simulink model "RoboBoatVU_2014_Bacchus"  (R2014a)
settings: Solver=FixedStepDiscrete  StartTime=0.0  StopTime=inf  FixedStep=.1  RelTol=1e-3
undefined symbols (not defined in the file): Com1, Com2, Com3, Com4, DiscIntNeverNeededParam, RGB24, standard
libraries: visiontextngfix x51, simulink x44, xpcseriallib x15, dspmtrx3 x14, speedgoatlib_IO102 x3, slrtlib x2, visionstatistics x2, dspstat3 x2, dspindex x2, xpcvideousblib x2, xpcvideoutillib x2, speedgoatlib x1
(part 2 of 5)

== matlab function RoboBoatVU_2014_Bacchus/Main FSM/Obstacle Navigation1/Enter Gate/Gate 1 (Red & White)/Distance ==
  data: Distance output; DesiredGPS input; GPSLat input; GPSLong input
function Distance  = DistCalc(DesiredGPS, GPSLat, GPSLong)

%Written by Anderson Lebbad on July 22, 2013
%Last Edited:

%Orients the boat towards a target GPS point before approaching it.
%This is done to keep the approach angle minimal, so the approach
%algorithm does not circle the target and never reach it.

%Parse input GPS and convert angles to radians
CurLat = (floor(GPSLat/100)+mod(GPSLat,100)/60)*pi/180;
CurLong = (floor(GPSLong/100)+mod(GPSLong,100)/60)*pi/180;
DesLat = (floor(DesiredGPS(1)/100)+mod(DesiredGPS(1),100)/60)*pi/180;
DesLong = (floor(DesiredGPS(2)/100)+mod(DesiredGPS(2),100)/60)*pi/180;
%Difference between lats and longs
DiffLat = DesLat - CurLat;
MidLat = cos((CurLat + DesLat)/2);
DiffLong = DesLong - CurLong;
%Radius of the earth in meters
R = 6378137;

%Calculate distance using the great-circle distance formula
%Formula documented here:
%   http://www.movable-type.co.uk/scripts/latlong.html
% a = sin(DiffLat/2)^2+sin(DiffLong/2)^2*cos(CurLat)*cos(DesLat);
% c = 2*atan2(sqrt(a), sqrt(1-a));
% Distance = R*c;

%Calculating distance using Pythagora's
a = DiffLong*MidLat;
b = DiffLat;
Distance = R*sqrt(a^2+b^2);

== matlab function RoboBoatVU_2014_Bacchus/Main FSM/Obstacle Navigation1/Enter Gate/Gate 2 (White & White)/MATLAB Function ==
  data: Prob input; RPM output; ColorID input; Dist input; Ang input; CurrentHeading input; GPSLat input; GPSLong input; Timer input; DesiredHeading output; gateGPS output
function [RPM,DesiredHeading,gateGPS] = navigation(Prob,ColorID,Dist,Ang,CurrentHeading,GPSLat,GPSLong,Timer)

% Function performs one buoy navigation through the start speed gates. If
% no buoys are found by the LIDAR/Vision assembly then an incremented
% turning algorithm is executed to turn by 10 degrees per increment up to 
% 90 degrees either way of the inital heading

% Written by Edward Zhu


persistent LockHeading TimeLastFound Counter Turn TurnInc gateLat gateLong

if isempty(LockHeading) && isempty(TimeLastFound) && isempty(Counter) && isempty(Turn) && isempty(TurnInc)
    LockHeading = CurrentHeading;
    TimeLastFound = 0;
    Counter = 0;
    TurnInc = 30;
    Turn = TurnInc;
    gateLat = 0;
    gateLong = 0;
end
Distance = Dist/100;
BoatWidth = 0.75;
Buffer = atan(2*BoatWidth/Distance);

RedOffset = Ang + Buffer;
WhiteOffset = Ang - Buffer;

R = 6378137;

CurLat = (floor(GPSLat/100)+mod(GPSLat,100)/60)*pi/180;
CurLong = (ceil(GPSLong/100)-mod(-GPSLong,100)/60)*pi/180;

gateHeading = (mod(CurrentHeading - Ang, 360))*pi/180;

if ColorID == 1 && Prob > 0.9
    DesiredHeading = mod(CurrentHeading - RedOffset, 360);
    RPM = 2000;
    GateFound = 1;
    TimeLastFound = Timer;
    gateLat =  asin(sin(CurLat)*cos(Distance/R) + cos(CurLat)*sin(Distance/R)*cos(gateHeading))*180/pi;
    gateLong = (CurLong + atan2(sin(gateHeading)*sin(Distance/R)*cos(CurLat),cos(Distance/R)-sin(CurLat)*sin(gateLat)))*180/pi;
elseif ColorID == 2 && Prob > 0.9
    DesiredHeading = mod(CurrentHeading - WhiteOffset, 360);
    RPM = 2000;
    GateFound = 1;
    TimeLastFound = Timer;
    gateLat =  asin(sin(CurLat)*cos(Distance/R) + cos(CurLat)*sin(Distance/R)*cos(gateHeading))*180/pi;
    gateLong = (CurLong + atan2(sin(gateHeading)*sin(Distance/R)*cos(CurLat),cos(Distance/R)-sin(CurLat)*sin(gateLat)))*180/pi;
else
    DesiredHeading = CurrentHeading;
    RPM = 0;
    GateFound = 0;
end

gateGPS = [gateLat gateLong];
TimeNoBuoys = Timer - TimeLastFound;

if GateFound == 0 && TimeNoBuoys > 15
    RPM = 0;
    DesiredHeading = mod(LockHeading - Turn, 360);
    HeadingDiff = DesiredHeading - CurrentHeading;
    gateGPS = [gateLat gateLong];
    
    if HeadingDiff > 180
        HeadingDiff = HeadingDiff - 360;
    elseif HeadingDiff < -180
        HeadingDiff = HeadingDiff + 360;
    end
    
    if HeadingDiff < 3
        Counter = Counter + 1;
    else
        Counter = 0;
    end
    
    if Counter >= 15
        Turn = Turn + TurnInc;
        Counter = 0;
        if abs(Turn) > 90
            TurnInc = -TurnInc;
        end
    end
end

== matlab function RoboBoatVU_2014_Bacchus/Main FSM/Communication/Docking Bay Comm/MATLAB Function ==
  data: requestNumOut output; CP input; requestNumIn input; Finished output
function [requestNumOut, Finished] = requestSender(CP, requestNumIn)

if CP < 1
    requestNumOut = requestNumIn;
    Finished = 0;
else
    requestNumOut = 0;
    Finished = 1;
end
end

== matlab function RoboBoatVU_2014_Bacchus/Main FSM/Color Sequence Detection/Report/MATLAB Function ==
  data: requestNumOut output; CP input; requestNumIn input; Finished output
function [requestNumOut, Finished] = requestSender(CP, requestNumIn)

if CP < 1
    requestNumOut = requestNumIn;
    Finished = 0;
else
    requestNumOut = 0;
    Finished = 1;
end

== matlab function RoboBoatVU_2014_Bacchus/Main FSM/Obstacle Navigation1/GPS: Center/Approach/Desired Heading and Distance ==
  data: Distance output; DesiredGPS input; DesiredHeading output; GPSLat input; GPSLong input
function [Distance, DesiredHeading] = Approach(DesiredGPS, GPSLat, GPSLong)

%Written by Anderson Lebbad on July 22, 2013
%Last Edited: Edward Zhu July 5, 2014

%Edit:
% Switched from great-circle distance formula to equirectangular approx and
%used mod for desired heading
% Changed calculation to use positve lat and negative long

%Orients the boat towards a target GPS point before approaching it.
%This is done to keep the approach angle minimal, so the approach
%algorithm does not circle the target and never reach it.

%Parse input GPS and convert angles to radians
CurLat = (floor(GPSLat/100)+mod(GPSLat,100)/60)*pi/180;
CurLong = (ceil(GPSLong/100)-mod(-GPSLong,100)/60)*pi/180;
DesLat = (floor(DesiredGPS(1)/100)+mod(DesiredGPS(1),100)/60)*pi/180;
DesLong = (ceil(DesiredGPS(2)/100)-mod(-DesiredGPS(2),100)/60)*pi/180;

%Difference between lats and longs
DiffLat = DesLat - CurLat;
MidLat = cos((CurLat + DesLat)/2);
DiffLong = DesLong - CurLong;

%Radius of the earth in meters
R = 6378137;

%Calculate distance using the great-circle distance formula
%Formula documented here:
%   http://www.movable-type.co.uk/scripts/latlong.html
% a = sin(DiffLat/2)^2+sin(DiffLong/2)^2*cos(CurLat)*cos(DesLat);
% c = 2*atan2(sqrt(a), sqrt(1-a));
% Distance = R*c;

%Calculating distance using equirectangular approximation since distances
%concerned are very small
a = DiffLong*MidLat;
b = DiffLat;
Distance = R*sqrt(a^2+b^2);

%Calculate initial bearing - formula documented here: 
%   http://www.movable-type.co.uk/scripts/latlong.html
y = sin(DiffLong)*cos(DesLat);
x = cos(CurLat)*sin(DesLat)-sin(CurLat)*cos(DesLat)*cos(DiffLong);
DesiredHeading = mod(atan2(y, x)*180/pi + 360, 360);

== matlab function RoboBoatVU_2014_Bacchus/Main FSM/Obstacle Navigation1/Obstacle Navigation/GPS: Bee Line/Approach/Obstacle Distance ==
  data: ColorID input; ObstDist output; DodgeStart output; Dist input
function [ObstDist, DodgeStart] = obstDist(ColorID,Dist)

%Written by Edward Zhu
%Last Edited by:

ObstDist = Dist / 100;

% if ColorID == 5 || ColorID == 6
    if ObstDist <= 3
        DodgeStart = 1;
    else
        DodgeStart = 0;
    end
% else
%     DodgeStart = 0;
% end

== matlab function RoboBoatVU_2014_Bacchus/Sensors/Serial In/Decode Compass/Correct Heading Angle Magnetic to True North/Magnetic to True North Conversion ==
  data: HeadingM input; HeadingT output; MagDec input
function HeadingT = fcn(HeadingM,MagDec)
% This function corrects the compass heading reading from magnetic north to
% true north

% Magnetic declination at Villanova is -12.116 degrees (West)
% Magnetic declination at competition site is -10.877 degrees (West)

% Current physical orientation of the compass is 0 degrees north measuring
% heading CCW, the standard for measuring heading is 0 degrees north 
% measuring CW. Therefore, first the heading is corrected to true heading
% by adding the declination. Then the heading is negated and added to 360
% in order to match with the standard measurment.

HeadingT = mod((HeadingM - MagDec) + 360, 360);

== matlab function RoboBoatVU_2014_Bacchus/Main FSM/Obstacle Navigation1/Obstacle Navigation/MATLAB Function ==
  data: dodgeIncomplete input; dodgeStart input; taskSelector output; dodgeEn output; GPSEn output
function [taskSelector, dodgeEn, GPSEn]  = obstNavEnabler(dodgeIncomplete, dodgeStart)

GPSEn = 0;
dodgeEn = 0;

if  dodgeStart == 1 || dodgeIncomplete == 1
    dodgeEn = 1;
    taskSelector = 1;
else
    GPSEn = 1;
    taskSelector = 2;
end

== matlab function RoboBoatVU_2014_Bacchus/Main FSM/Main Task Option/Message Composer ==
  data: taskStrInit input; taskStrAdj output
function taskStrAdj = composeMessage(taskStrInit)
%Written by Anderson Lebbad on August 9, 2013
%Last Edited: Edward Zhu on June 2, 2014

%This function adjusts the length of a vector to a set value by filling
%the remaining space with 0's. This is necessary for data store objects
%that have a fixed size for the memory allocation, but a variable length
%input.

%Length of message packet
strLength = 8;

%Size of text in message
taskStrLength = size(taskStrInit,1);

%Pad end of text with zeros
taskStrAdj = [taskStrInit' zeros(1,strLength-taskStrLength)];

== system RoboBoatVU_2014_Bacchus/Main FSM/Communication/Docking Bay Comm ==
  Sensors : Inport
  RGB image : Inport  Port=2
  Enable : EnablePort  ShowOutputPort=on
  Annotate Task : visiontextngfix/Insert Text  inputType=Obsolete  theText='Docking Bay Request...'  getTextLocFrom=Specify via dialog  textLoc=[10 10]  getTextColorFrom=Specify via dialog  textColor=[0 0 255]  getTextIntensityFrom=Specify via dialog  textIntensity=0  getTextOpacityFrom=Specify via dialog  textOpacity=1.0  dummyVar2=0  dummyVar3=0  dummyVar4=0  imagePorts=One multidimensional signal  isInputTransposed=off  fontFace=LucidaSansRegular  dummyVar1=0  blockFontSize=12  antiAliased=on
  Annotate Task1 : visiontextngfix/Insert Text  inputType=Obsolete  theText='CP: %f'  getTextLocFrom=Specify via dialog  textLoc=[10 20]  getTextColorFrom=Specify via dialog  textColor=[0 0 255]  getTextIntensityFrom=Specify via dialog  textIntensity=0  getTextOpacityFrom=Specify via dialog  textOpacity=1.0  dummyVar2=0  dummyVar3=0  dummyVar4=0  imagePorts=One multidimensional signal  isInputTransposed=off  fontFace=LucidaSansRegular  dummyVar1=0  blockFontSize=12  antiAliased=on
  Bus Selector : BusSelector  OutputSignals=Serial In.Compass.Heading,Serial In.Comms.CP,Serial In.Comms.Dat1
  Compare To Constant : simulink/Logic and Bit Operations/Compare To Constant  relop=>=  const=15  OutDataTypeStr=boolean
  Constant : Constant  Value=2
  Data Store Write : DataStoreWrite  DataStoreName=dockBay
  Data Type Conversion : DataTypeConversion  OutDataTypeStr=double
  Discrete-Time Integrator : DiscreteIntegrator  SampleTime=0.1  ICPrevOutput=DiscIntNeverNeededParam  ICPrevScaledInput=DiscIntNeverNeededParam
  Logical Operator : Logic  Operator=OR  AllPortsSameDT=off  OutDataTypeStr=boolean
  MATLAB Function : MATLAB Function  TreatAsAtomicUnit=on
  Output Heirarchy : Subsystem
  Outputs : Outport
  wires:
  Sensors/1 -> Bus Selector/1, Output Heirarchy/3(Sensors)  "Sensors"
  Bus Selector/1 -> Output Heirarchy/2(Desired Heading)  "<Heading>"
  RGB image/1 -> Annotate Task/1
  Annotate Task/1 -> Annotate Task1/1
  Output Heirarchy/1(Outputs) -> Outputs/1
  Enable/1 -> Discrete-Time Integrator/1
  Discrete-Time Integrator/1 -> Compare To Constant/1
  Data Type Conversion/1 -> Output Heirarchy/5(Task Finished)
  Bus Selector/2 -> Annotate Task1/2, MATLAB Function/1(CP)  "<CP>"
  Constant/1 -> MATLAB Function/2(requestNumIn)
  MATLAB Function/1(requestNumOut) -> Output Heirarchy/4(Request Number)
  Logical Operator/1 -> Data Type Conversion/1
  MATLAB Function/2(Finished) -> Logical Operator/1
  Compare To Constant/1 -> Logical Operator/2
  Annotate Task1/1 -> Output Heirarchy/1(Annotated Image)
  Bus Selector/3 -> Data Store Write/1  "<Dat1>"

== system RoboBoatVU_2014_Bacchus/Main FSM/Communication/Obst Gate Comm ==
  Sensors : Inport
  RGB image : Inport  Port=2
  Enable : EnablePort  ShowOutputPort=on
  Annotate Task : visiontextngfix/Insert Text  inputType=Obsolete  theText='Obstacle Navigation Request...'  getTextLocFrom=Specify via dialog  textLoc=[10 10]  getTextColorFrom=Specify via dialog  textColor=[0 0 255]  getTextIntensityFrom=Specify via dialog  textIntensity=0  getTextOpacityFrom=Specify via dialog  textOpacity=1.0  dummyVar2=0  dummyVar3=0  dummyVar4=0  imagePorts=One multidimensional signal  isInputTransposed=off  fontFace=LucidaSansRegular  dummyVar1=0  blockFontSize=12  antiAliased=on
  Annotate Task1 : visiontextngfix/Insert Text  inputType=Obsolete  theText='CP: %f'  getTextLocFrom=Specify via dialog  textLoc=[10 20]  getTextColorFrom=Specify via dialog  textColor=[0 0 255]  getTextIntensityFrom=Specify via dialog  textIntensity=0  getTextOpacityFrom=Specify via dialog  textOpacity=1.0  dummyVar2=0  dummyVar3=0  dummyVar4=0  imagePorts=One multidimensional signal  isInputTransposed=off  fontFace=LucidaSansRegular  dummyVar1=0  blockFontSize=12  antiAliased=on
  Bus Selector : BusSelector  OutputSignals=Serial In.Comms.CP,Serial In.Comms.Dat1,Serial In.Comms.Dat2,Serial In.Compass.Heading
  Compare To Constant : simulink/Logic and Bit Operations/Compare To Constant  relop=>=  const=15  OutDataTypeStr=boolean
  Constant : Constant
  Data Store Write : DataStoreWrite  DataStoreName=enterGate
  Data Store Write1 : DataStoreWrite  DataStoreName=exitGate
  Data Type Conversion : DataTypeConversion  OutDataTypeStr=double
  Discrete-Time Integrator : DiscreteIntegrator  SampleTime=0.1  ICPrevOutput=DiscIntNeverNeededParam  ICPrevScaledInput=DiscIntNeverNeededParam
  Logical Operator : Logic  Operator=OR  AllPortsSameDT=off  OutDataTypeStr=boolean
  MATLAB Function : MATLAB Function  TreatAsAtomicUnit=on
  Output Heirarchy : Subsystem
  Outputs : Outport
  Finished : Outport  Port=2
  wires:
  Sensors/1 -> Bus Selector/1, Output Heirarchy/3(Sensors)  "Sensors"
  Bus Selector/4 -> Output Heirarchy/2(Desired Heading)  "<Heading>"
  RGB image/1 -> Annotate Task/1
  Output Heirarchy/1(Outputs) -> Outputs/1
  Enable/1 -> Discrete-Time Integrator/1
  Discrete-Time Integrator/1 -> Compare To Constant/1
  Annotate Task/1 -> Annotate Task1/1
  Bus Selector/1 -> MATLAB Function/1(CP), Annotate Task1/2  "<CP>"
  Annotate Task1/1 -> Output Heirarchy/1(Annotated Image)
  Data Type Conversion/1 -> Finished/1
  MATLAB Function/1(requestNumOut) -> Output Heirarchy/4(Request Number)
  Constant/1 -> MATLAB Function/2(requestNumIn)
  Logical Operator/1 -> Data Type Conversion/1
  MATLAB Function/2(Finished) -> Logical Operator/1
  Compare To Constant/1 -> Logical Operator/2
  Bus Selector/2 -> Data Store Write/1  "<Dat1>"
  Bus Selector/3 -> Data Store Write1/1  "<Dat2>"

== system RoboBoatVU_2014_Bacchus/Main FSM/Communication/Output Reassign ==
  Outputs in : Inport
  Bus Selector : BusSelector  OutputSignals=Task Finished,Output Signals
  Outputs : Outport
  Finished : Outport  Port=2
  wires:
  Outputs in/1 -> Bus Selector/1
  Bus Selector/1 -> Finished/1  "<Task Finished>"
  Bus Selector/2 -> Outputs/1  "<Output Signals>"

== system RoboBoatVU_2014_Bacchus/Main FSM/Docking/Output Heirarchy ==
  Annotated Image : Inport
  Desired Heading : Inport  Port=2
  Sensors : Inport  Port=3
  Request Number : Inport  Port=4
  Bus Creator : BusCreator  Inputs=2
  Bus Creator1 : BusCreator  Inputs=3
  Bus Creator2 : BusCreator  Inputs=2
  Bus Creator3 : BusCreator  Inputs=6
  Bus Creator4 : BusCreator  Inputs=2
  C1 : Constant  Value=0
  C2 : Constant  Value=0
  C3 : Constant  Value=0
  LPTask : Constant  Value=0
  Latitude : Constant  Value=0
  Longitude : Constant  Value=0
  RPM Desired : Constant  Value=0
  Outputs : Outport
  wires:
  RPM Desired/1 -> Bus Creator/1  "RPM"
  Bus Creator/1 -> Bus Creator1/1  "Control Signals"
  Bus Creator3/1 -> Bus Creator2/1  "Comms Panda"
  Request Number/1 -> Bus Creator3/1  "Request Number"
  Latitude/1 -> Bus Creator3/2  "Latitude"
  Longitude/1 -> Bus Creator3/3  "Longitude"
  C1/1 -> Bus Creator3/4  "C1"
  LPTask/1 -> Bus Creator2/2  "LIDAR Panda"
  Desired Heading/1 -> Bus Creator/2  "Desired Heading"
  Bus Creator1/1 -> Bus Creator4/1  "Outputs"
  Annotated Image/1 -> Bus Creator1/3  "Annotated Image"
  Sensors/1 -> Bus Creator4/2  "Sensors"
  Bus Creator4/1 -> Outputs/1  "Output Signals"
  Bus Creator2/1 -> Bus Creator1/2  "Serial Outputs"
  C2/1 -> Bus Creator3/5  "C2"
  C3/1 -> Bus Creator3/6  "C3"

== system RoboBoatVU_2014_Bacchus/Main FSM/Initialization1/Output Heirarchy ==
  Annotated Image : Inport
  Desired Heading : Inport  Port=2
  Sensors : Inport  Port=3
  Request Number : Inport  Port=4
  Bus Creator : BusCreator  Inputs=2
  Bus Creator1 : BusCreator  Inputs=3
  Bus Creator2 : BusCreator  Inputs=2
  Bus Creator3 : BusCreator  Inputs=6
  Bus Creator4 : BusCreator  Inputs=2
  C1 : Constant  Value=0
  C2 : Constant  Value=0
  C3 : Constant  Value=0
  LPTask : Constant  Value=0
  Latitude : Constant  Value=0
  Longitude : Constant  Value=0
  RPM Desired : Constant  Value=0
  Outputs : Outport
  wires:
  RPM Desired/1 -> Bus Creator/1  "RPM"
  Bus Creator/1 -> Bus Creator1/1  "Control Signals"
  Bus Creator3/1 -> Bus Creator2/1  "Comms Panda"
  Request Number/1 -> Bus Creator3/1  "Request Number"
  Latitude/1 -> Bus Creator3/2  "Latitude"
  Longitude/1 -> Bus Creator3/3  "Longitude"
  C1/1 -> Bus Creator3/4  "C1"
  LPTask/1 -> Bus Creator2/2  "LIDAR Panda"
  Desired Heading/1 -> Bus Creator/2  "Desired Heading"
  Bus Creator1/1 -> Bus Creator4/1  "Outputs"
  Annotated Image/1 -> Bus Creator1/3  "Annotated Image"
  Sensors/1 -> Bus Creator4/2  "Sensors"
  Bus Creator4/1 -> Outputs/1  "Output Signals"
  Bus Creator2/1 -> Bus Creator1/2  "Serial Outputs"
  C2/1 -> Bus Creator3/5  "C2"
  C3/1 -> Bus Creator3/6  "C3"

== system RoboBoatVU_2014_Bacchus/Main FSM/Obstacle Navigation/Dodge ==
  Sensors : Inport
  RGB image : Inport  Port=2
  Enable : EnablePort  ShowOutputPort=on
  Bus Selector1 : BusSelector  OutputSignals=Serial In.Compass.Heading,Serial In.Buoy Info.Distance,Serial In.Buoy Info.Angle
  Constant : Constant  Value=0
  Constant1 : Constant  Value=2
  Data Store Write : DataStoreWrite  DataStoreName=dodgeStart
  Discrete-Time Integrator : DiscreteIntegrator  SampleTime=0.1  ICPrevOutput=DiscIntNeverNeededParam  ICPrevScaledInput=DiscIntNeverNeededParam
  Insert Text : visiontextngfix/Insert Text  inputType=Obsolete  theText='Dodge'  getTextLocFrom=Specify via dialog  textLoc=[1 1]  getTextColorFrom=Specify via dialog  textColor=[0 0 0]  getTextIntensityFrom=Specify via dialog  textIntensity=0  getTextOpacityFrom=Specify via dialog  textOpacity=1.0  dummyVar2=0  dummyVar3=0  dummyVar4=0  imagePorts=One multidimensional signal  isInputTransposed=off  fontFace=LucidaSansRegular  dummyVar1=0  blockFontSize=12  antiAliased=on
  Insert Text1 : visiontextngfix/Insert Text  inputType=Obsolete  theText='Obstacle Distance: %f'  getTextLocFrom=Specify via dialog  textLoc=[10 70]  getTextColorFrom=Specify via dialog  textColor=[255 0 0]  getTextIntensityFrom=Specify via dialog  textIntensity=0  getTextOpacityFrom=Specify via dialog  textOpacity=1.0  dummyVar2=0  dummyVar3=0  dummyVar4=0  imagePorts=One multidimensional signal  isInputTransposed=off  fontFace=LucidaSansRegular  dummyVar1=0  blockFontSize=12  antiAliased=on
  Nav Logic : MATLAB Function  TreatAsAtomicUnit=on
  Output Heirarchy : Subsystem
  Unit Delay1 : UnitDelay  InitialCondition=1  SampleTime=-1
  Outputs : Outport
  Dodge Incomplete : Outport  Port=2
  wires:
  RGB image/1 -> Insert Text/1
  Sensors/1 -> Output Heirarchy/2(Sensors), Bus Selector1/1
  Bus Selector1/1 -> Nav Logic/1(CurrentHeading)  "<Heading>"
  Enable/1 -> Discrete-Time Integrator/1
  Discrete-Time Integrator/1 -> Nav Logic/4(Timer)
  Constant1/1 -> Nav Logic/5(Timeout)
  Nav Logic/4(DodgeIncomplete) -> Dodge Incomplete/1
  Insert Text/1 -> Insert Text1/1
  Nav Logic/1(ObstDist) -> Insert Text1/2
  Output Heirarchy/1(Outputs) -> Outputs/1
  Constant/1 -> Unit Delay1/1
  Unit Delay1/1 -> Data Store Write/1
  Insert Text1/1 -> Output Heirarchy/1(Annotated Image)
  Bus Selector1/2 -> Nav Logic/2(Dist)  "<Distance>"
  Bus Selector1/3 -> Nav Logic/3(Ang)  "<Angle>"
  Nav Logic/2(RPM) -> Output Heirarchy/3(RPM)
  Nav Logic/3(DesiredHeading) -> Output Heirarchy/4(Desired Heading)

== system RoboBoatVU_2014_Bacchus/Main FSM/Obstacle Navigation/GPS: Bee Line ==
  Sensors : Inport
  RGB image : Inport  Port=2
  Enable : EnablePort
  Approach : Subsystem  TreatAsAtomicUnit=on
  Data Store Write : DataStoreWrite  DataStoreName=dodgeStart
  GPS Enabler : MATLAB Function  TreatAsAtomicUnit=on
  GPS Selector : MultiPortSwitch  Inputs=2
  Orient : Subsystem  TreatAsAtomicUnit=on
  Unit Delay : UnitDelay  SampleTime=-1
  Unit Delay1 : UnitDelay  SampleTime=-1
  Outputs : Outport
  wires:
  Sensors/1 -> Orient/1(Sensors), Approach/1(Sensors)
  GPS Enabler/2(OrientEnable) -> Orient/Enable
  GPS Enabler/3(ApproachEnable) -> Approach/Enable
  Orient/2(Finished) -> Unit Delay/1
  Orient/1(Outputs) -> GPS Selector/2
  Approach/1(Outputs) -> GPS Selector/3
  GPS Enabler/1(GPSMode) -> GPS Selector/1
  Unit Delay/1 -> GPS Enabler/1(Finished)
  RGB image/1 -> Orient/2(RGB image), Approach/2(RGB image)
  Approach/2(Dodge Start) -> Unit Delay1/1
  Unit Delay1/1 -> Data Store Write/1
  GPS Selector/1 -> Outputs/1

== system RoboBoatVU_2014_Bacchus/Main FSM/Obstacle Navigation/Output Reassign ==
  Outputs in : Inport
  Bus Assignment : BusAssignment  Commented=on  AssignedSignals=Task Finished
  Bus Selector : BusSelector  OutputSignals=Task Finished,Output Signals
  Constant : Constant  Commented=on  Value=0
  Outputs : Outport
  Finished : Outport  Port=2
  wires:
  Bus Selector/1 -> Finished/1  "<Task Finished>"
  Outputs in/1 -> Bus Selector/1
  Constant/1 -> Bus Assignment/2
  Bus Selector/2 -> Outputs/1  "<Output Signals>"

== system RoboBoatVU_2014_Bacchus/Main FSM/Obstacle Navigation1/Communication ==
  Sensors : Inport
  RGB Image : Inport  Port=2
  Enable : EnablePort  ShowOutputPort=on
  Bus Selector : BusSelector  OutputSignals=Serial In.Compass.Heading
  Compare To Constant : simulink/Logic and Bit Operations/Compare To Constant  relop=>=  const=5  OutDataTypeStr=boolean
  Constant : Constant  Value=3
  Constant1 : Constant  Value=3
  Data Store Write : DataStoreWrite  DataStoreName=enterGate
  Data Store Write1 : DataStoreWrite  DataStoreName=exitGate
  Data Type Conversion : DataTypeConversion  OutDataTypeStr=double
  Discrete-Time Integrator : DiscreteIntegrator  SampleTime=0.1  ICPrevOutput=DiscIntNeverNeededParam  ICPrevScaledInput=DiscIntNeverNeededParam
  Insert Text : visiontextngfix/Insert Text  inputType=Obsolete  theText='Communication1'  getTextLocFrom=Specify via dialog  textLoc=[1 1]  getTextColorFrom=Specify via dialog  textColor=[0 0 0]  getTextIntensityFrom=Specify via dialog  textIntensity=0  getTextOpacityFrom=Specify via dialog  textOpacity=1.0  dummyVar2=0  dummyVar3=0  dummyVar4=0  imagePorts=One multidimensional signal  isInputTransposed=off  fontFace=LucidaSansRegular  dummyVar1=0  blockFontSize=12  antiAliased=on
  Output Heirarchy1 : Subsystem
  Outputs : Outport
  Finished : Outport  Port=2
  wires:
  Constant/1 -> Data Store Write/1
  Constant1/1 -> Data Store Write1/1
  Insert Text/1 -> Output Heirarchy1/3(Annotated Image)
  RGB Image/1 -> Insert Text/1
  Sensors/1 -> Bus Selector/1, Output Heirarchy1/2(Sensors)
  Bus Selector/1 -> Output Heirarchy1/1(Desired Heading)  "<Heading>"
  Enable/1 -> Discrete-Time Integrator/1
  Discrete-Time Integrator/1 -> Compare To Constant/1
  Data Type Conversion/1 -> Finished/1
  Compare To Constant/1 -> Data Type Conversion/1
  Output Heirarchy1/1(Outputs) -> Outputs/1

== system RoboBoatVU_2014_Bacchus/Main FSM/Obstacle Navigation1/Enter Gate ==
  Sensors : Inport
  RGB Image : Inport  Port=2
  Enable : EnablePort
  Data Store Read : DataStoreRead  DataStoreName=enterGate
  Gate 1 (Red & White) : Subsystem  TreatAsAtomicUnit=on
  Gate 2 (White & White) : Subsystem  TreatAsAtomicUnit=on
  Gate 3 (White & Green) : Subsystem  TreatAsAtomicUnit=on
  MATLAB Function : MATLAB Function  TreatAsAtomicUnit=on
  Multiport Switch : MultiPortSwitch
  Output Reassign : Subsystem
  Outputs : Outport
  Finished : Outport  Port=2
  wires:
  Data Store Read/1 -> MATLAB Function/1(gateID)
  MATLAB Function/2(gate1En) -> Gate 1 (Red & White)/Enable
  MATLAB Function/3(gate2En) -> Gate 2 (White & White)/Enable
  MATLAB Function/4(gate3En) -> Gate 3 (White & Green)/Enable
  RGB Image/1 -> Gate 1 (Red & White)/2(RGB image), Gate 2 (White & White)/2(RGB image), Gate 3 (White & Green)/2(RGB image)
  Sensors/1 -> Gate 1 (Red & White)/1(Sensors), Gate 2 (White & White)/1(Sensors), Gate 3 (White & Green)/1(Sensors)
  Gate 1 (Red & White)/1(Outputs) -> Multiport Switch/2
  Gate 2 (White & White)/1(Outputs) -> Multiport Switch/3
  Gate 3 (White & Green)/1(Outputs) -> Multiport Switch/4
  MATLAB Function/1(outputSelector) -> Multiport Switch/1
  Multiport Switch/1 -> Output Reassign/1(Outputs in)
  Output Reassign/1(Outputs) -> Outputs/1
  Output Reassign/2(Finished) -> Finished/1

== system RoboBoatVU_2014_Bacchus/Main FSM/Obstacle Navigation1/Exit Gate ==
  Sensors : Inport
  RGB Image : Inport  Port=2
  Enable : EnablePort
  Data Store Read : DataStoreRead  DataStoreName=exitGate
  Gate 1 (Red & White) : Subsystem  TreatAsAtomicUnit=on
  Gate 2 (White & White) : Subsystem  TreatAsAtomicUnit=on
  Gate 3 (White & Green) : Subsystem  TreatAsAtomicUnit=on
  MATLAB Function : MATLAB Function  TreatAsAtomicUnit=on
  Multiport Switch : MultiPortSwitch
  Outputs : Outport
  wires:
  Data Store Read/1 -> MATLAB Function/1(gateID)
  MATLAB Function/2(gate1En) -> Gate 1 (Red & White)/Enable
  MATLAB Function/3(gate2En) -> Gate 2 (White & White)/Enable
  MATLAB Function/4(gate3En) -> Gate 3 (White & Green)/Enable
  RGB Image/1 -> Gate 1 (Red & White)/2(RGB image), Gate 2 (White & White)/2(RGB image), Gate 3 (White & Green)/2(RGB image)
  Sensors/1 -> Gate 1 (Red & White)/1(Sensors), Gate 2 (White & White)/1(Sensors), Gate 3 (White & Green)/1(Sensors)
  Gate 1 (Red & White)/1(Outputs) -> Multiport Switch/2
  Gate 2 (White & White)/1(Outputs) -> Multiport Switch/3
  Gate 3 (White & Green)/1(Outputs) -> Multiport Switch/4
  MATLAB Function/1(outputSelector) -> Multiport Switch/1
  Multiport Switch/1 -> Outputs/1

== system RoboBoatVU_2014_Bacchus/Main FSM/Obstacle Navigation1/GPS: Center ==
  Sensors : Inport
  RGB image : Inport  Port=2
  Enable : EnablePort
  Approach : Subsystem  TreatAsAtomicUnit=on
  GPS Enabler : MATLAB Function  TreatAsAtomicUnit=on
  GPS Selector : MultiPortSwitch  Inputs=2
  Orient : Subsystem  TreatAsAtomicUnit=on
  Output Reassign : Subsystem
  Unit Delay : UnitDelay  SampleTime=-1
  Outputs : Outport
  Finished : Outport  Port=2
  wires:
  Output Reassign/1(Outputs) -> Outputs/1
  Output Reassign/2(Finished) -> Finished/1
  Sensors/1 -> Approach/1(Sensors), Orient/1(Sensors)
  GPS Enabler/2(OrientEnable) -> Orient/Enable
  GPS Enabler/3(ApproachEnable) -> Approach/Enable
  Orient/2(Finished) -> Unit Delay/1
  Orient/1(Outputs) -> GPS Selector/2
  Approach/1(Outputs) -> GPS Selector/3
  GPS Enabler/1(GPSMode) -> GPS Selector/1
  Unit Delay/1 -> GPS Enabler/1(Finished)
  GPS Selector/1 -> Output Reassign/1(Outputs in)
  RGB image/1 -> Approach/2(RGB image), Orient/2(RGB image)

== system RoboBoatVU_2014_Bacchus/Main FSM/Obstacle Navigation1/Obstacle Navigation ==
  Sensors : Inport
  RGB Image : Inport  Port=2
  Enable : EnablePort
  Data Store Read : DataStoreRead  DataStoreName=dodgeStart
  Dodge : Subsystem  TreatAsAtomicUnit=on
  GPS: Bee Line : Subsystem  TreatAsAtomicUnit=on
  MATLAB Function : MATLAB Function  TreatAsAtomicUnit=on
  Multiport Switch : MultiPortSwitch  Inputs=2
  Output Reassign : Subsystem
  Unit Delay : UnitDelay  SampleTime=-1
  Outputs : Outport
  Finished : Outport  Port=2
  wires:
  MATLAB Function/3(GPSEn) -> GPS: Bee Line/Enable
  Sensors/1 -> GPS: Bee Line/1(Sensors), Dodge/1(Sensors)
  RGB Image/1 -> GPS: Bee Line/2(RGB image), Dodge/2(RGB image)
  MATLAB Function/2(dodgeEn) -> Dodge/Enable
  Dodge/1(Outputs) -> Multiport Switch/2
  GPS: Bee Line/1(Outputs) -> Multiport Switch/3
  MATLAB Function/1(taskSelector) -> Multiport Switch/1
  Dodge/2(Dodge Incomplete) -> Unit Delay/1  "Dodge Incomplete"
  Data Store Read/1 -> MATLAB Function/2(dodgeStart)
  Unit Delay/1 -> MATLAB Function/1(dodgeIncomplete)
  Multiport Switch/1 -> Output Reassign/1(Outputs in)
  Output Reassign/1(Outputs) -> Outputs/1
  Output Reassign/2(Finished) -> Finished/1

== system RoboBoatVU_2014_Bacchus/Main FSM/Obstacle Navigation1/Output Reassign ==
  Outputs in : Inport
  Bus Selector : BusSelector  OutputSignals=Task Finished,Output Signals
  Outputs : Outport
  Finished : Outport  Port=2
  wires:
  Outputs in/1 -> Bus Selector/1
  Bus Selector/1 -> Finished/1  "<Task Finished>"
  Bus Selector/2 -> Outputs/1  "<Output Signals>"

== system RoboBoatVU_2014_Bacchus/Main FSM/Obstacle Navigation1/Task Option1 ==
  note: Obstacle Nav Options
  Message Composer : MATLAB Function  TreatAsAtomicUnit=on
  Obstacle Nav : Constant  Value=uint8('12345678')  SampleTime=0.1
  Option : Outport
  wires:
  Obstacle Nav/1 -> Message Composer/1(taskStrInit)
  Message Composer/1(taskStrAdj) -> Option/1

== system RoboBoatVU_2014_Bacchus/Main FSM/Obstacle Navigation2/Output Heirarchy ==
  Annotated Image : Inport
  Desired Heading : Inport  Port=2
  Sensors : Inport  Port=3
  Request Number : Inport  Port=4
  Bus Creator : BusCreator  Inputs=2
  Bus Creator1 : BusCreator  Inputs=3
  Bus Creator2 : BusCreator  Inputs=2
  Bus Creator3 : BusCreator  Inputs=6
  Bus Creator4 : BusCreator  Inputs=2
  C1 : Constant  Value=0
  C2 : Constant  Value=0
  C3 : Constant  Value=0
  LPTask : Constant  Value=0
  Latitude : Constant  Value=0
  Longitude : Constant  Value=0
  RPM Desired : Constant  Value=0
  Outputs : Outport
  wires:
  RPM Desired/1 -> Bus Creator/1  "RPM"
  Bus Creator/1 -> Bus Creator1/1  "Control Signals"
  Bus Creator3/1 -> Bus Creator2/1  "Comms Panda"
  Request Number/1 -> Bus Creator3/1  "Request Number"
  Latitude/1 -> Bus Creator3/2  "Latitude"
  Longitude/1 -> Bus Creator3/3  "Longitude"
  C1/1 -> Bus Creator3/4  "C1"
  LPTask/1 -> Bus Creator2/2  "LIDAR Panda"
  Desired Heading/1 -> Bus Creator/2  "Desired Heading"
  Bus Creator1/1 -> Bus Creator4/1  "Outputs"
  Annotated Image/1 -> Bus Creator1/3  "Annotated Image"
  Sensors/1 -> Bus Creator4/2  "Sensors"
  Bus Creator4/1 -> Outputs/1  "Output Signals"
  Bus Creator2/1 -> Bus Creator1/2  "Serial Outputs"
  C2/1 -> Bus Creator3/5  "C2"
  C3/1 -> Bus Creator3/6  "C3"

== system RoboBoatVU_2014_Bacchus/Main FSM/RCHold/Output Heirarchy ==
  Desired Heading : Inport
  Annotated Image : Inport  Port=2
  Sensors : Inport  Port=3
  Bus Creator : BusCreator  Inputs=2
  Bus Creator1 : BusCreator  Inputs=3
  Bus Creator2 : BusCreator  Inputs=2
  Bus Creator3 : BusCreator  Inputs=6
  Bus Creator4 : BusCreator  Inputs=2
  C1 : Constant  Value=0
  C2 : Constant  Value=0
  C3 : Constant  Value=0
  LPTask : Constant  Value=0
  Latitude : Constant  Value=0
  Longitude : Constant  Value=0
  RPM Desired : Constant  Value=0
  Request Number : Constant  Value=0
  Outputs : Outport
  wires:
  RPM Desired/1 -> Bus Creator/1  "RPM"
  Bus Creator/1 -> Bus Creator1/1  "Control Signals"
  Bus Creator3/1 -> Bus Creator2/1  "Comms Panda"
  Request Number/1 -> Bus Creator3/1  "Request Number"
  Latitude/1 -> Bus Creator3/2  "Latitude"
  Longitude/1 -> Bus Creator3/3  "Longitude"
  C1/1 -> Bus Creator3/4  "C1"
  LPTask/1 -> Bus Creator2/2  "LIDAR Panda"
  Desired Heading/1 -> Bus Creator/2  "Desired Heading"
  Bus Creator1/1 -> Bus Creator4/1  "Outputs"
  Annotated Image/1 -> Bus Creator1/3  "Annotated Image"
  Sensors/1 -> Bus Creator4/2  "Sensors"
  Bus Creator4/1 -> Outputs/1  "Output Signals"
  Bus Creator2/1 -> Bus Creator1/2  "Serial Outputs"
  C2/1 -> Bus Creator3/5  "C2"
  C3/1 -> Bus Creator3/6  "C3"

== system RoboBoatVU_2014_Bacchus/Main FSM/Return to Start/Output Heirarchy ==
  Annotated Image : Inport
  Desired Heading : Inport  Port=2
  Sensors : Inport  Port=3
  Bus Creator : BusCreator  Inputs=2
  Bus Creator1 : BusCreator  Inputs=3
  Bus Creator2 : BusCreator  Inputs=2
  Bus Creator3 : BusCreator  Inputs=6
  Bus Creator4 : BusCreator  Inputs=2
  C1 : Constant  Value=0
  C2 : Constant  Value=0
  C3 : Constant  Value=0
  LPTask : Constant  Value=0
  Latitude : Constant  Value=0
  Longitude : Constant  Value=0
  RPM Desired : Constant  Value=0
  Request Number : Constant  Value=0
  Outputs : Outport
  wires:
  RPM Desired/1 -> Bus Creator/1  "RPM"
  Bus Creator/1 -> Bus Creator1/1  "Control Signals"
  Bus Creator3/1 -> Bus Creator2/1  "Comms Panda"
  Request Number/1 -> Bus Creator3/1  "Request Number"
  Latitude/1 -> Bus Creator3/2  "Latitude"
  Longitude/1 -> Bus Creator3/3  "Longitude"
  C1/1 -> Bus Creator3/4  "C1"
  LPTask/1 -> Bus Creator2/2  "LIDAR Panda"
  Desired Heading/1 -> Bus Creator/2  "Desired Heading"
  Bus Creator1/1 -> Bus Creator4/1  "Outputs"
  Annotated Image/1 -> Bus Creator1/3  "Annotated Image"
  Sensors/1 -> Bus Creator4/2  "Sensors"
  Bus Creator4/1 -> Outputs/1  "Output Signals"
  Bus Creator2/1 -> Bus Creator1/2  "Serial Outputs"
  C2/1 -> Bus Creator3/5  "C2"
  C3/1 -> Bus Creator3/6  "C3"

== system RoboBoatVU_2014_Bacchus/Main FSM/Start Speed Gate/Buoy Decisions ==
  Sensors : Inport
  RGB image : Inport  Port=2
  Red + Green : Inport  Port=3
  Timer : Inport  Port=4
  Annotate Image : Subsystem
  Bus Selector : BusSelector  OutputSignals=Serial In.Compass.Heading
  Bus Selector1 : BusSelector  OutputSignals=Red BBox,Green BBox,Red Centroid,Green Centroid
  Nav Logic : MATLAB Function  TreatAsAtomicUnit=on
  Read : DataStoreRead  DataStoreName=Course
  Annotated Image : Outport
  RPM : Outport  Port=2
  Desired Heading : Outport  Port=3
  wires:
  RGB image/1 -> Annotate Image/1(RGB image)
  Red + Green/1 -> Bus Selector1/1
  Annotate Image/1(Annotated Image) -> Annotated Image/1
  Bus Selector1/1 -> Annotate Image/2(Red BBox), Nav Logic/2(RedBBox)  "<Red BBox>"
  Bus Selector1/2 -> Annotate Image/3(Green BBox), Nav Logic/3(GreenBBox)  "<Green BBox>"
  Bus Selector1/3 -> Nav Logic/4(RedCentroid)  "<Red Centroid>"
  Bus Selector1/4 -> Nav Logic/5(GreenCentroid)  "<Green Centroid>"
  Bus Selector/1 -> Nav Logic/1(Compass)  "<Heading>"
  Sensors/1 -> Bus Selector/1
  Nav Logic/1(RedDist) -> Annotate Image/4(Red Dist)
  Nav Logic/2(GreenDist) -> Annotate Image/5(Green Dist)
  Nav Logic/3(RPM) -> RPM/1
  Nav Logic/4(DesiredHeading) -> Desired Heading/1
  Read/1 -> Nav Logic/6(Course)
  Timer/1 -> Nav Logic/7(Timer)

== system RoboBoatVU_2014_Bacchus/Main FSM/Start Speed Gate/Output Heirarchy ==
  Sensors : Inport
  Annotated Image : Inport  Port=2
  RPM : Inport  Port=3
  Desired Heading : Inport  Port=4
  Bus Creator : BusCreator  Inputs=2
  Bus Creator1 : BusCreator  Inputs=3
  Bus Creator2 : BusCreator  Inputs=2
  Bus Creator3 : BusCreator  Inputs=6
  Bus Creator4 : BusCreator  Inputs=2
  C1 : Constant  Value=0
  C2 : Constant  Value=0
  C3 : Constant  Value=0
  LPTask : Constant
  Latitude : Constant  Value=0
  Longitude : Constant  Value=0
  Request Number : Constant  Value=0
  Outputs : Outport
  wires:
  Bus Creator/1 -> Bus Creator1/1  "Control Signals"
  Bus Creator3/1 -> Bus Creator2/1  "Comms Panda"
  Request Number/1 -> Bus Creator3/1  "Request Number"
  Latitude/1 -> Bus Creator3/2  "Latitude"
  Longitude/1 -> Bus Creator3/3  "Longitude"
  C1/1 -> Bus Creator3/4  "C1"
  LPTask/1 -> Bus Creator2/2  "LIDAR Panda"
  Bus Creator1/1 -> Bus Creator4/1  "Outputs"
  Annotated Image/1 -> Bus Creator1/3  "Annotated Image"
  Sensors/1 -> Bus Creator4/2  "Sensors"
  Bus Creator4/1 -> Outputs/1  "Output Signals"
  Bus Creator2/1 -> Bus Creator1/2  "Serial Outputs"
  C2/1 -> Bus Creator3/5  "C2"
  C3/1 -> Bus Creator3/6  "C3"
  RPM/1 -> Bus Creator/1  "RPM"
  Desired Heading/1 -> Bus Creator/2  "Desired Heading"

== system RoboBoatVU_2014_Bacchus/Main FSM/Start Speed Gate/Start Speed Gate Detection ==
  RGB : Inport
  Bus Creator : BusCreator
  Green Detection : Subsystem
  Red Detection : Subsystem
  S-Function : S-Function  FunctionName=rgbtohsv_int_sfun  EnableBusSupport=off
  Red + Green : Outport
  wires:
  RGB/1 -> S-Function/1
  S-Function/1 -> Green Detection/1(HSV), Red Detection/1(HSV)
  Red Detection/1(Red Centroid) -> Bus Creator/1  "Red Centroid"
  Red Detection/2(Red BBox) -> Bus Creator/2  "Red BBox"
  Green Detection/1(Green Centroid) -> Bus Creator/3  "Green Centroid"
  Green Detection/2(Green BBox) -> Bus Creator/4  "Green BBox"
  Bus Creator/1 -> Red + Green/1

== system RoboBoatVU_2014_Bacchus/Main FSM/Termination/Output Heirarchy ==
  Annotated Image : Inport
  Desired Heading : Inport  Port=2
  Sensors : Inport  Port=3
  Bus Creator : BusCreator  Inputs=2
  Bus Creator1 : BusCreator  Inputs=3
  Bus Creator2 : BusCreator  Inputs=2
  Bus Creator3 : BusCreator  Inputs=6
  Bus Creator4 : BusCreator  Inputs=2
  C1 : Constant  Value=0
  C2 : Constant  Value=0
  C3 : Constant  Value=0
  LPTask : Constant  Value=0
  Latitude : Constant  Value=0
  Longitude : Constant  Value=0
  RPM Desired : Constant  Value=0
  Request Number : Constant  Value=10
  Outputs : Outport
  wires:
  RPM Desired/1 -> Bus Creator/1  "RPM"
  Bus Creator/1 -> Bus Creator1/1  "Control Signals"
  Bus Creator3/1 -> Bus Creator2/1  "Comms Panda"
  Request Number/1 -> Bus Creator3/1  "Request Number"
  Latitude/1 -> Bus Creator3/2  "Latitude"
  Longitude/1 -> Bus Creator3/3  "Longitude"
  C1/1 -> Bus Creator3/4  "C1"
  LPTask/1 -> Bus Creator2/2  "LIDAR Panda"
  Desired Heading/1 -> Bus Creator/2  "Desired Heading"
  Bus Creator1/1 -> Bus Creator4/1  "Outputs"
  Annotated Image/1 -> Bus Creator1/3  "Annotated Image"
  Sensors/1 -> Bus Creator4/2  "Sensors"
  Bus Creator4/1 -> Outputs/1  "Output Signals"
  Bus Creator2/1 -> Bus Creator1/2  "Serial Outputs"
  C2/1 -> Bus Creator3/5  "C2"
  C3/1 -> Bus Creator3/6  "C3"

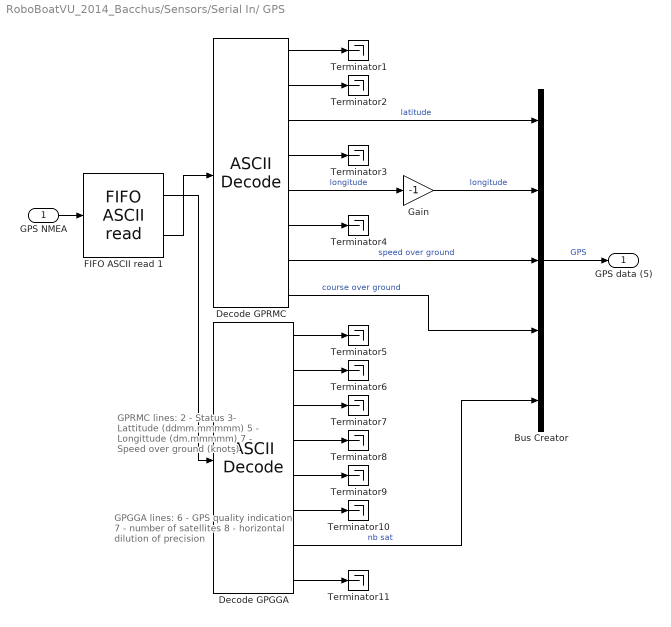
== system RoboBoatVU_2014_Bacchus/Sensors/Serial In/ GPS ==
  note: GPGGA lines:
      | 6 - GPS quality indication
      | 7 - number of satellites
      | 8 - horizontal dilution of precision
  note: GPRMC lines:
      | 2 - Status
      | 3- Lattitude (ddmm.mmmmm)
      | 5 - Longittude (dm.mmmmm)
      | 7 - Speed over ground (knots)
  GPS NMEA : Inport
  Bus Creator : BusCreator  Inputs=5
  Decode GPGGA : xpcseriallib/ASCII Decode   format=$GPGGA,%d,%f,%c%f,%c%f,%f,%f  nvars=8  vartypes={ }
  Decode GPRMC : xpcseriallib/ASCII Decode   format=$GPRMC,%f,%c%f,%c%f,%c%f,%f  nvars=8  vartypes={ }
  FIFO ASCII read 1 : xpcseriallib/FIFO ASCII read   header={'$GPGGA','$GPRMC'}  term=[13 10]  hold=Zero output if no new data  enable=off  maxsize=1024  outputtype=8 bit uint null terminated  sampletime=-1
  Gain : Gain  Gain=-1
  Terminator{1..11} (11 alike) : Terminator
  GPS data (5) : Outport
  wires:
  Decode GPRMC/1 -> Terminator1/1
  Decode GPRMC/7 -> Bus Creator/3  "speed over ground"
  Decode GPRMC/5 -> Gain/1  "longitude"
  Decode GPRMC/3 -> Bus Creator/1  "latitude"
  GPS NMEA/1 -> FIFO ASCII read 1/1
  FIFO ASCII read 1/1 -> Decode GPGGA/1
  FIFO ASCII read 1/2 -> Decode GPRMC/1
  Decode GPRMC/8 -> Bus Creator/4  "course over ground"
  Decode GPGGA/7 -> Bus Creator/5  "nb sat"
  Decode GPRMC/2 -> Terminator2/1
  Decode GPRMC/4 -> Terminator3/1
  Decode GPRMC/6 -> Terminator4/1
  Decode GPGGA/1 -> Terminator5/1
  Decode GPGGA/2 -> Terminator6/1
  Decode GPGGA/3 -> Terminator7/1
  Decode GPGGA/4 -> Terminator8/1
  Decode GPGGA/5 -> Terminator9/1
  Decode GPGGA/6 -> Terminator10/1
  Decode GPGGA/8 -> Terminator11/1
  Bus Creator/1 -> GPS data (5)/1  "GPS"
  Gain/1 -> Bus Creator/2  "longitude"

== system RoboBoatVU_2014_Bacchus/Sensors/Serial In/Arduino Due ==
  Arduino Due In : Inport
  ASCII Decode 1 : xpcseriallib/ASCII Decode   format=H1:%04d,H2:%04d,PD:%04d,PA:%04d\r\n  nvars=4  vartypes={'double'}
  Bus Creator : BusCreator
  "FIFO ASCII read " : xpcseriallib/FIFO ASCII read   header={'H1:'}  term=[13 10]  hold=Zero output if no new data  enable=off  maxsize=1024  outputtype=8 bit uint null terminated  sampletime=0.1
  Arduino Due Out : Outport
  wires:
  "FIFO ASCII read "/1 -> ASCII Decode 1/1
  Arduino Due In/1 -> "FIFO ASCII read "/1
  ASCII Decode 1/1 -> Bus Creator/1  "Mag 1"
  ASCII Decode 1/2 -> Bus Creator/2  "Mag 2"
  ASCII Decode 1/3 -> Bus Creator/3  "Pinger Dist"
  ASCII Decode 1/4 -> Bus Creator/4  "Pinger Ang"
  Bus Creator/1 -> Arduino Due Out/1  "Arduino Messages"

== system RoboBoatVU_2014_Bacchus/Sensors/Serial In/Communication Panda ==
  Comm Panda In : Inport
  ASCII Decode 6 : xpcseriallib/ASCII Decode   format=CP:%d Dat1:%d Dat2:%d \r\n  nvars=3  vartypes={}
  Bus Creator4 : BusCreator  Inputs=3
  FIFO ASCII read 1 : xpcseriallib/FIFO ASCII read   header={'CP:'}  term=[13 10]  hold=Zero output if no new data  enable=off  maxsize=1024  outputtype=8 bit uint null terminated  sampletime=0.1
  Comm Panda Out : Outport
  wires:
  Comm Panda In/1 -> FIFO ASCII read 1/1
  FIFO ASCII read 1/1 -> ASCII Decode 6/1
  ASCII Decode 6/1 -> Bus Creator4/1  "CP"
  ASCII Decode 6/2 -> Bus Creator4/2  "Dat1"
  Bus Creator4/1 -> Comm Panda Out/1  "Comms"
  ASCII Decode 6/3 -> Bus Creator4/3  "Dat2"

== system RoboBoatVU_2014_Bacchus/Sensors/Serial In/Decode Compass ==
  note: Status Field can be one of the following:
      | L = low alarm
      | M= low warning
      | N = Normal
      | O = High Warning
      | P = High Alarm
      | C = Tuning analog circuit
  note: Compas NMEA- Raw data from the Compass
  Compass NMEA : Inport
  "ASCII Decode " : xpcseriallib/ASCII Decode   format=$PTNTHPR,%f,%c%f,%c%f,%c  nvars=7  vartypes={ }
  Bus Creator : BusCreator  Inputs=3
  Correct Heading Angle Magnetic to True North : Subsystem
  "FIFO ASCII read " : xpcseriallib/FIFO ASCII read   header={'$PTNTHPR'}  term=[13 10]  hold=Zero output if no new data  enable=off  maxsize=64  outputtype=8 bit uint null terminated  sampletime=-1
  Terminator{,1..3} (4 alike) : Terminator
  Compass data (3) : Outport
  wires:
  "FIFO ASCII read "/1 -> "ASCII Decode "/1
  Compass NMEA/1 -> "FIFO ASCII read "/1
  "ASCII Decode "/2 -> Terminator/1
  "ASCII Decode "/4 -> Terminator1/1
  "ASCII Decode "/6 -> Terminator2/1
  "ASCII Decode "/7 -> Terminator3/1
  Bus Creator/1 -> Compass data (3)/1  "Compass"
  "ASCII Decode "/3 -> Bus Creator/2  "Pitch"
  "ASCII Decode "/5 -> Bus Creator/3  "Roll"
  "ASCII Decode "/1 -> Correct Heading Angle Magnetic to True North/1(Heading Mag)  "Heading"
  Correct Heading Angle Magnetic to True North/1(Heading True) -> Bus Creator/1  "Heading"

== system RoboBoatVU_2014_Bacchus/Sensors/Serial In/LIDAR Panda ==
  LIDAR Panda In : Inport
  ASCII Decode 2 : xpcseriallib/ASCII Decode   format=Prob:%f Color:%d Dist:%d Ang:%d \r\n  nvars=4  vartypes={}
  Bus Creator1 : BusCreator
  "FIFO ASCII read " : xpcseriallib/FIFO ASCII read   header={'Prob:'}  term=[13 10]  hold=Zero output if no new data  enable=off  maxsize=1024  outputtype=8 bit uint null terminated  sampletime=0.1
  LIDAR Panda Out : Outport
  wires:
  LIDAR Panda In/1 -> "FIFO ASCII read "/1
  Bus Creator1/1 -> LIDAR Panda Out/1  "Buoy Info"
  ASCII Decode 2/2 -> Bus Creator1/2  "Color ID"
  ASCII Decode 2/1 -> Bus Creator1/1  "Probability"
  ASCII Decode 2/3 -> Bus Creator1/3  "Distance"
  ASCII Decode 2/4 -> Bus Creator1/4  "Angle"
  "FIFO ASCII read "/1 -> ASCII Decode 2/1

== system RoboBoatVU_2014_Bacchus/Sinks/actuators/analog output ==
  Compass Heading : Inport
  Control Signals : Inport  Port=2
  Analog output : speedgoatlib_IO102/Analog output  id=1  channels=[1,2,3,4]  range=2  ts=0.1  pciSlot=-1
  Ground : Ground
  Subsystem : Subsystem
  wires:
  Subsystem/1(Propulsion) -> Analog output/1
  Subsystem/2(Steering) -> Analog output/2
  Control Signals/1 -> Subsystem/2(Control Signals)
  Compass Heading/1 -> Subsystem/1(Compass Heading)
  Ground/1 -> Analog output/4, Analog output/3

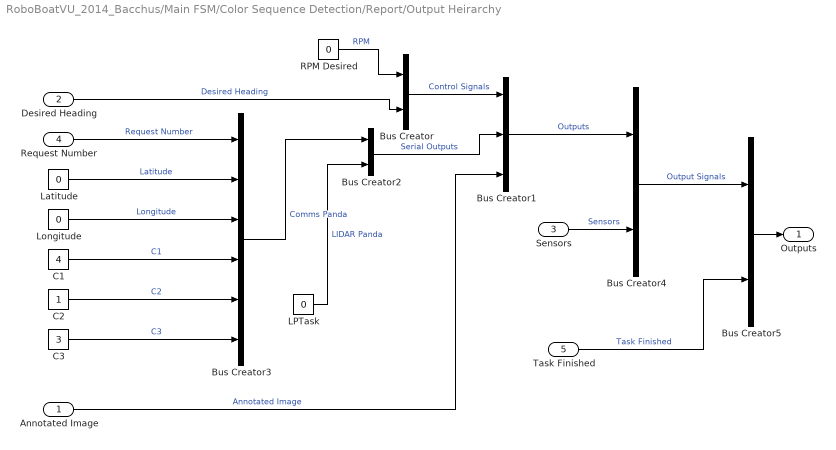
== system RoboBoatVU_2014_Bacchus/Main FSM/Color Sequence Detection/Report/Output Heirarchy ==
  Annotated Image : Inport
  Desired Heading : Inport  Port=2
  Sensors : Inport  Port=3
  Request Number : Inport  Port=4
  Task Finished : Inport  Port=5
  Bus Creator{,2,4..5} (4 alike) : BusCreator  Inputs=2
  Bus Creator1 : BusCreator  Inputs=3
  Bus Creator3 : BusCreator  Inputs=6
  C1 : Constant  Value=4
  C2 : Constant
  C3 : Constant  Value=3
  LPTask : Constant  Value=0
  Latitude : Constant  Value=0
  Longitude : Constant  Value=0
  RPM Desired : Constant  Value=0
  Outputs : Outport
  wires:
  RPM Desired/1 -> Bus Creator/1  "RPM"
  Bus Creator/1 -> Bus Creator1/1  "Control Signals"
  Bus Creator3/1 -> Bus Creator2/1  "Comms Panda"
  Request Number/1 -> Bus Creator3/1  "Request Number"
  Latitude/1 -> Bus Creator3/2  "Latitude"
  Longitude/1 -> Bus Creator3/3  "Longitude"
  C1/1 -> Bus Creator3/4  "C1"
  LPTask/1 -> Bus Creator2/2  "LIDAR Panda"
  Desired Heading/1 -> Bus Creator/2  "Desired Heading"
  Bus Creator1/1 -> Bus Creator4/1  "Outputs"
  Annotated Image/1 -> Bus Creator1/3  "Annotated Image"
  Sensors/1 -> Bus Creator4/2  "Sensors"
  Bus Creator4/1 -> Bus Creator5/1  "Output Signals"
  Bus Creator2/1 -> Bus Creator1/2  "Serial Outputs"
  C2/1 -> Bus Creator3/5  "C2"
  C3/1 -> Bus Creator3/6  "C3"
  Task Finished/1 -> Bus Creator5/2  "Task Finished"
  Bus Creator5/1 -> Outputs/1

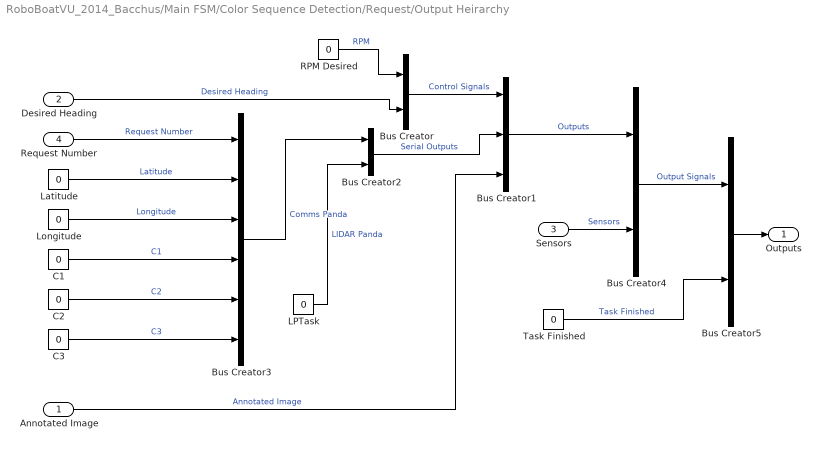
== system RoboBoatVU_2014_Bacchus/Main FSM/Color Sequence Detection/Request/Output Heirarchy ==
  Annotated Image : Inport
  Desired Heading : Inport  Port=2
  Sensors : Inport  Port=3
  Request Number : Inport  Port=4
  Bus Creator{,2,4..5} (4 alike) : BusCreator  Inputs=2
  Bus Creator1 : BusCreator  Inputs=3
  Bus Creator3 : BusCreator  Inputs=6
  C1 : Constant  Value=0
  C2 : Constant  Value=0
  C3 : Constant  Value=0
  LPTask : Constant  Value=0
  Latitude : Constant  Value=0
  Longitude : Constant  Value=0
  RPM Desired : Constant  Value=0
  Task Finished : Constant  Value=0
  Outputs : Outport
  wires:
  RPM Desired/1 -> Bus Creator/1  "RPM"
  Bus Creator/1 -> Bus Creator1/1  "Control Signals"
  Bus Creator3/1 -> Bus Creator2/1  "Comms Panda"
  Request Number/1 -> Bus Creator3/1  "Request Number"
  Latitude/1 -> Bus Creator3/2  "Latitude"
  Longitude/1 -> Bus Creator3/3  "Longitude"
  C1/1 -> Bus Creator3/4  "C1"
  LPTask/1 -> Bus Creator2/2  "LIDAR Panda"
  Desired Heading/1 -> Bus Creator/2  "Desired Heading"
  Bus Creator1/1 -> Bus Creator4/1  "Outputs"
  Annotated Image/1 -> Bus Creator1/3  "Annotated Image"
  Sensors/1 -> Bus Creator4/2  "Sensors"
  Bus Creator4/1 -> Bus Creator5/1  "Output Signals"
  Bus Creator2/1 -> Bus Creator1/2  "Serial Outputs"
  C2/1 -> Bus Creator3/5  "C2"
  C3/1 -> Bus Creator3/6  "C3"
  Task Finished/1 -> Bus Creator5/2  "Task Finished"
  Bus Creator5/1 -> Outputs/1

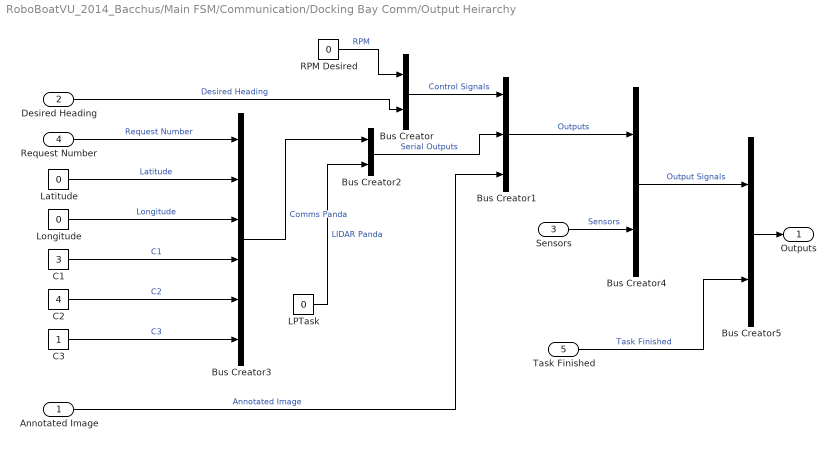
== system RoboBoatVU_2014_Bacchus/Main FSM/Communication/Docking Bay Comm/Output Heirarchy ==
  Annotated Image : Inport
  Desired Heading : Inport  Port=2
  Sensors : Inport  Port=3
  Request Number : Inport  Port=4
  Task Finished : Inport  Port=5
  Bus Creator{,2,4..5} (4 alike) : BusCreator  Inputs=2
  Bus Creator1 : BusCreator  Inputs=3
  Bus Creator3 : BusCreator  Inputs=6
  C1 : Constant  Value=3
  C2 : Constant  Value=4
  C3 : Constant
  LPTask : Constant  Value=0
  Latitude : Constant  Value=0
  Longitude : Constant  Value=0
  RPM Desired : Constant  Value=0
  Outputs : Outport
  wires:
  RPM Desired/1 -> Bus Creator/1  "RPM"
  Bus Creator/1 -> Bus Creator1/1  "Control Signals"
  Bus Creator3/1 -> Bus Creator2/1  "Comms Panda"
  Request Number/1 -> Bus Creator3/1  "Request Number"
  Latitude/1 -> Bus Creator3/2  "Latitude"
  Longitude/1 -> Bus Creator3/3  "Longitude"
  C1/1 -> Bus Creator3/4  "C1"
  LPTask/1 -> Bus Creator2/2  "LIDAR Panda"
  Desired Heading/1 -> Bus Creator/2  "Desired Heading"
  Bus Creator1/1 -> Bus Creator4/1  "Outputs"
  Annotated Image/1 -> Bus Creator1/3  "Annotated Image"
  Sensors/1 -> Bus Creator4/2  "Sensors"
  Bus Creator4/1 -> Bus Creator5/1  "Output Signals"
  Bus Creator2/1 -> Bus Creator1/2  "Serial Outputs"
  C2/1 -> Bus Creator3/5  "C2"
  C3/1 -> Bus Creator3/6  "C3"
  Task Finished/1 -> Bus Creator5/2  "Task Finished"
  Bus Creator5/1 -> Outputs/1
